simulink model "testboard_UW_GNCDE"  (R2019a)
settings: Solver=FixedStepAuto  StartTime=0.0  StopTime=100  FixedStep=0.05  RelTol=1e-3
values from neighbouring files (symbols this model uses):
  D = zeros(6,3)    [MPCController_test.m]
undefined symbols (not defined in the file or in its folder): Continuous, DiscIntNeverNeededParam, MPCController_test, MPCController_testq, Time
libraries: aerolibutil x23, sharedtransform x5, simulink_extras x4, simulink x4, sharedutil x4, ephemeris x3, sb_quatrans x3, ATV_cowell_plus_tides x2, FO_frame_q x2, FO_ang_vel x2, reference_frame_inv_change x2, sb_qua2con x2
(part 1 of 3)
settings Model: Creator=Jeong miri  LastModifiedBy=Jeong miri
settings SolverCC: AlgebraicLoopSolver=LineSearch
settings DataIOCC: ReturnWorkspaceOutputs=off
settings DebuggingCC: ArithmeticOperatorsInVariantConditions=warning
settings SFSimCC: SimUseLocalCustomCode=off
settings RTWCC: RTWUseLocalCustomCode=off

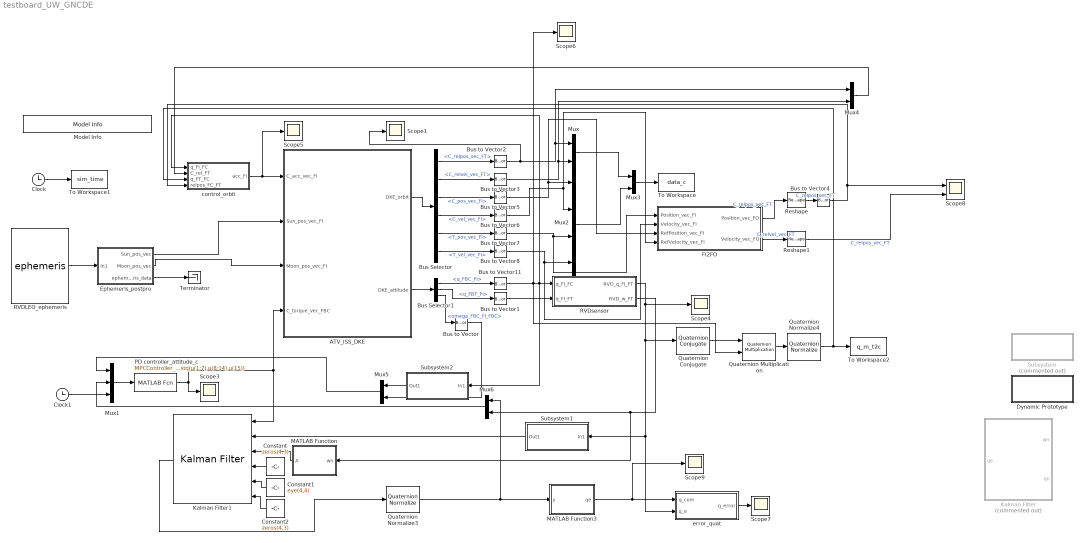
== system testboard_UW_GNCDE ==
  ATV_ISS_DKE : Subsystem
  Bus Selector : BusSelector  OutputSignals=C_relpos_vec_FT,C_relvel_vec_FT,C_pos_vec_FI,C_vel_vec_FI,T_pos_vec_FI,T_vel_vec_FI
  Bus Selector1 : BusSelector  OutputSignals=q_FBC_FI,q_FBT_FI,omega_FBC_FI_FBC
  Bus to Vector{,1..8,11} (10 alike) : BusToVector
  Clock : Clock
  Clock1 : Clock
  Constant : Constant  Value=zeros(4,3)
  Constant1 : Constant  Value=eye(4,4)
  Constant2 : Constant  Value=zeros(4,3)
  Dynamic Prototype : Subsystem
  Ephemeris_postpro : Subsystem
  FI2FO : Subsystem  AncestorBlock=FI_2_FO/FI2FO
  Kalman Filter : Subsystem  Commented=on
  Kalman Filter1 : ctrlSharedLib/Kalman Filter  TimeDomain=Continuous-Time  UseCurrentEstimator=on  ModelSource=Input port  ModelSourceVariable=ss(0.95,1,1,0,1)  A=0.95  B=zeros(3,3)  C=eye(3,3)  D=zeros(3,3)  NumberOfStates=4  NumberOfInputs=3  NumberOfOutputs=4  InitialEstimateSource=Dialog  X0=[0.2685;-0.1449;0.1277;0.9437]  P0=1*eye(4)  UseK=off  UseGH=on  NumberOfProcessNoiseInputs=1  G=eye(4)  TimeInvariantG=on  H=eye(4)  TimeInvariantH=on  Q=(0.25^2)*eye(4)  TimeInvariantQ=on  R=5*eye(4)  TimeInvariantR=on  N=0  TimeInvariantN=on  AddInputPort=on  AddEnablePort=off  OutputEstimatedY=off  OutputP=off  Ts=0.05
      settings: SourceProductBaseCode=CT
  MATLAB Function : MATLAB Function  TreatAsAtomicUnit=on
  MATLAB Function3 : MATLAB Function  TreatAsAtomicUnit=on
  Model Info : simulink/Model-Wide Utilities/Model Info  Frame=on  DisplayStringWithTags=using matlab quaternion formation [1 0 0 0]  HorizontalTextAlignment=Center  LeftAlignmentValue=0.5
  Mux{,3..6} (5 alike) : Mux  Inputs=2
  Mux1 : Mux  Inputs=3
  Mux2 : Mux
  PD controller_attitude_c : MATLABFcn  MATLABFcn=MPCController_testq(u(1:7),u(8:14),u(15))  OutputDimensions=3
  Quaternion Conjugate : aerolibutil/Quaternion Conjugate
      settings: SourceProductName=Aerospace Blockset  SourceProductBaseCode=AE
  Quaternion Multiplication : aerolibutil/Quaternion Multiplication
  Quaternion Normalize3 : sharedutil/Quaternion Normalize  aMode=aMode
      settings: SourceProductName=Aerospace Blockset  SourceProductBaseCode=AE
  Quaternion Normalize4 : sharedutil/Quaternion Normalize  aMode=aMode
      settings: SourceProductName=Aerospace Blockset  SourceProductBaseCode=AE
  RVDLEO_ephemeris : ephemeris/ephemeris  DiagCtrlNo=6  Ini_option=Specify via M-File  InitFileName=D:\GNCDE\working_folder\RVDLEO_ephemeris_init.m  NewFile_Action=Cancel  OldFile_Action=Cancel  InitStatus=on  Ini_Epoch=5479  Enable_Body=[0 0 1 0 0 0 0 0 0 1 1 0 0]  chbycf=struct('EAR',[5474.0194925278993 5479.6117378982699 10 -19525649687.250961 -7242210690.4189663 12591507.829688819 712045.59300004842 -4605.6625453254146 219.47025289226869 7.4245048250737691 -1.279428349516061 0.125436043400523 -0.0071881873469209229 -0.001528338274485566 133532390146.9698 -921020264.59608769 -81156138.833497182 137258.18726933541 1958.221018748188 -226.45025145371531 19.04438678085301 -0.47565199325122492 -0.029635518085251819 0.013715571797866871 -0.0013136744370657459 57865920681.460564 -399022325.11280107 -35186655.777805582 54285.092220920029 985.14747069403722 -69.615781388512403 6.5400659798170437 -0.19345718613262849 -0.0066813954077421999 0.0044218866970717188 -0.00045458987392305651;5479.6117378982699 5485.4983119723438 10 -34254548400.29591 -7477438242.8778076 23337177.440669671 787909.51370320341 -101.42364834386559 199.86116801645741 -13.88804847021297 -0.4553042858772216 0.078328146498667775 0.0059646795681814746 -0.0010337031674248431 130955284596.13721 -1663171194.276058 -87925053.51922065 179251.61568709169 1388.5831853938671 132.30829303924551 9.512894879359461 -1.0347453844758461 -0.041263310503606522 0.0060887801194377117 0.00052000420269988521 56749025379.978554 -720980819.72698534 -38162991.360703968 77270.96408691231 1016.182799768875 49.167254600843748 2.8008634855034802 -0.35644771507836259 -0.011929311143635459 0.0022070878965816838 0.00014552259262877749;5485.4983119723438 5491.3848860464177 10 -48992679504.172363 -7252760915.1633511 32857451.614941169 801439.50634623843 1101.8143140951399 0.083647783492835262 3.9255766985739471 0.82019475446432044 -0.061798440081102357 -0.0061011152711196162 -0.0002389289953963916 126932773131.94701 -2357357426.2140589 -85540006.044280127 225511.99280920179 4182.0883657711947 88.662679826200574 -3.5479097565355282 0.81152795017696377 0.087199738015311973 -0.001151144659435246 -0.00017101715215852651 55004945370.370369 -1022217299.01609 -37102806.967740543 101895.7725987231 1971.0960883287471 28.70521160977616 -1.140951709445895 0.29051978417011931 0.027717464636542951 -0.00048242776422865698 -6.6677991161821385e-05;5491.3848860464177 5497.2714601204916 10 -63204647068.536743 -6951087933.3918591 42601686.903376661 824699.35841737944 1649.568043720418 -113.1790852983782 -41.022970444021972 -4.3406011450349444 0.070110924116653137 0.065367019483753938 0.0058988188212964988 121543214792.2896 -3029554236.4885492 -82357371.525249705 313732.82557588391 7943.5635573665686 408.7545116397921 18.400097415110199 -2.7277057817587891 -0.57221163955953691 -0.023246325824219521 0.0053081507161301267 52667973121.656143 -1313559489.3725569 -35666051.661055617 140488.6937452509 3215.2116641950338 132.83967448087751 5.289527673086579 -0.99991985655036242 -0.18955929431432891 -0.0063908294139869226 0.0019201328415656251;5497.2714601204916 5503.1580341945655 10 -76734737558.20166 -6570839091.8005066 52372771.716799781 772018.39095029037 -9944.6279617588989 -454.3681787485454 83.809068685693589 3.7919618233988972 -1.361770299950025 -0.026622466649221209 0.02451221935319188 114839053481.6221 -3670661103.2674298 -77618855.18230474 479784.41825950157 8682.2149673298591 -705.09161127909567 -38.806502953602752 9.8568103129389719 0.33397462270782607 -0.1701515171819207 -0.001317018702844246 49761592296.068863 -1591106544.9909611 -33607749.850501142 203098.60049911449 3197.4313406917122 -245.8172029376731 -11.19376541302562 3.3690215861258581 0.082996134226937704 -0.057386373093671249 7.2266565342218286e-05;5503.1580341945655 5509.3389369723436 10 -89729309568.452377 -6410491164.686923 67105136.35983476 721521.72513387376 -6928.6403657680194 432.94267085107168 -22.126363115256549 0.072413118060123932 0.30426059359918167 -0.049301053495564191 0.0024480440664662729 106675048463.05949 -4495427655.7620573 -78608325.722655028 606054.10099249275 -537.49477693948893 -26.30040712632232 24.681564052482059 -3.2413175158506959 0.26932602498584729 0.01063421455686926 -0.0051067636571243587 ...(+3004 chars)],'MOO',[5476.6131248693891 5481.114976721241 10 235949301.9451361 -139173673.45685661 -17032226.23224216 1771368.5992196151 71835.615581327787 -7540.910793108279 16.28634176898839 8.9471108610484045 -0.075149790432813265 0.073741168648467623 -0.0079991516308435175 252854781.41849309 127527608.8909824 -17736229.67664988 -1273994.0397991559 120401.39664943211 2097.2510112104869 -328.06212638437131 5.2330344486417859 -0.36780970941805829 0.045648828645552642 0.0054088502705201902 90789604.575848266 39511416.746048398 -6353352.9079350522 -382773.30564623408 41969.292298044027 508.7589280098282 -108.8642852811857 1.9853812338043171 -0.12726475804964901 0.017146034811725702 0.0016172965508710921;5481.114976721241 5486.0260878323525 10 -119281955.3483213 -194445073.75190681 8804733.5933451802 2314797.0242647119 -80112.933901338925 -5728.0071634057631 421.759363826666 -0.91181921354713247 -1.9488246940505889 -0.0084783699209460186 0.011503361945009101 333270850.53264862 -53856696.543870591 -24894022.82772788 876282.02549440751 131553.5833390374 -5694.0238152214242 -120.8246642842264 26.977974360037859 -0.069136334149162204 -0.1355218644754167 -0.00041516536287204377 109482735.19933949 -22556141.111693509 -8127972.0992596922 347532.41299178731 41893.033387395917 -2039.8857338279649 -29.532861950791968 8.9895693748721577 -0.069175183404102503 -0.0454504927427863 0.00013279297195722601;5486.0260878323525 5491.1418285730924 10 -368209659.5822103 -37272448.254160039 28966093.382118989 575792.99784778652 -147195.65970897651 -1320.7880421427931 -160.4890923653515 -24.126983670689832 1.796771915897017 0.1446034638555122 0.0033626189383728958 71454414.966571927 -191741260.26137051 -5312399.1746770367 2402447.2617379432 37282.834321171671 -3936.0102596018878 106.2381311707356 -27.158974243902669 -2.3056748101124969 0.036254948464378732 0.0017252666010675959 16003973.15075887 -65111328.583141513 -1125438.4316383279 814225.58604786242 8984.5804238699893 -1322.8460257668189 32.849456061550768 -9.6427815500062568 -0.72953118229025593 0.01518347286777523 0.00062416681064214065;5491.1418285730924 5495.8483100545745 10 -236519463.35481861 158989676.51849779 17929698.965212502 -1637619.3726077219 -148555.9306766433 -1013.984913001647 511.68040453812893 71.721969906101265 2.6806624200266191 -0.32312680059878268 -0.051766975946830517 -254997418.9626143 -114164435.1907489 19450237.914976511 1721414.0568385541 -68076.258331813486 -9423.4410594721303 -559.55193870543053 6.4195501401895942 5.5801097229978307 0.44785715250136943 -0.00073204452341000007 -90573889.219337761 -34836986.375739031 6887264.9110708293 538411.5582076998 -25810.146240520378 -3153.833007474484 -176.40199327653519 3.6184785576243348 1.918418425226208 0.14277676416418511 -0.001316420239122922;5495.8483100545745 5499.9409026471667 10 116401656.6447359 171813227.58897761 -7970534.7329276307 -1980863.751555094 25524.273659049239 11206.54795115962 167.1969016831396 -69.268389378915458 -3.278822889780431 0.47172691310630382 0.041157636499332413 -303323196.63847512 65757614.980408177 20611242.479798179 -543872.05192871974 -143426.6800424523 -92.085434493212006 813.24375163807758 25.531789254040699 -5.4093457119175339 -0.35587524108731272 0.036090681683312989 -99338439.864302963 25569036.202503979 6717133.6882401844 -223199.74185484409 -47253.39209144537 203.64275772509021 274.67240678849907 7.0777808184736957 -1.873842176894027 -0.1089760039254066 0.012906262764400741;5499.9409026471667 5504.2381248693891 10 335274982.68933171 31989042.783745591 -25328830.028744549 -162112.32263660929 178384.79872649111 -3587.6855037252139 -820.42089911496646 65.820233209958843 2.5672242334859812 -0.70311518487965996 0.016015888366578648 -42449594.014380872 180569964.27288741 3160527.406108255 -2220172.1798197869 10148.981021424101 11731.155453871979 -511.53838286409859 -48.826068979201182 6.727900076266061 0.040477776788079907 -0.062120147956740618 -7587826.408630427 61015956.372747831 534922.55756132503 ...(+4277 chars)],'SUN',[5478.8683078666654 5482.1318495333317 10 425902245.7615025 967998.27965419751 -617.75881662588279 0.45980846342291071 -0.0043364422167170577 -0.00020171772762461309 -1.225011122694448e-05 2.3865395757416262e-05 -2.9291117847822658e-07 -1.4546880485764169e-05 1.7380347169454301e-06 -108117502.82189821 1184470.971916039 573.98858879357738 0.81449435548467708 0.0123702264478636 0.00013669158135858479 3.0125458983458141e-06 2.1288618992704241e-05 -6.7756159307572082e-07 -1.403173841314433e-05 -1.857921382276252e-07 -69272546.646467105 487629.54570443952 253.7339345238355 0.32242200756521211 0.0068109215496674307 9.5519179459789061e-05 2.1833006097486991e-06 8.3557192063880096e-06 -2.1110260248094199e-07 -5.6051094059912039e-06 -2.0946789385142999e-07;5482.1318495333317 5485.3953911999988 10 427833316.66130322 963076.75062086084 -612.81277980640903 0.35080907664054523 -0.0098922992050331573 -0.00036380103125100522 3.4787407022091389e-05 -2.2510980377448619e-05 1.3232521644046419e-05 7.1238643550083942e-06 -2.365423327018569e-05 -105743935.5028107 1189105.5542703699 585.04217680491035 1.034374393213618 0.01494844902950113 0.0001128347597781029 4.9527524415888863e-05 -2.7796809432373019e-05 1.630835977050129e-05 8.7087311958026212e-06 -2.9201894700000078e-05 -68295244.023768201 489676.8979657052 258.32295275562421 0.4474318438385767 0.0087913834942875291 9.881859481749497e-05 2.0776569270259942e-05 -1.145538201128545e-05 6.7149878235458709e-06 3.5807508913316201e-06 -1.202574834275584e-05;5485.3953911999988 5488.6589328666651 10 429754578.667633 958187.74978908116 -609.83857615235684 0.1205345604510957 -0.01960343183724023 -0.0006127452198189477 -7.9062290558582653e-06 2.74258294033769e-05 1.048152071636293e-08 -3.1105645691112532e-06 -2.4413683898238059e-08 -103361001.81192879 1193839.709181759 598.92989905955869 1.281004497556963 0.015222974588530161 -0.00013087953892676479 -1.332699415056042e-05 3.3566256858805422e-05 2.6492958013671179e-08 -3.8929222441107083e-06 7.5831507774073641e-09 -67313804.871897265 491767.47291078261 264.58809424093681 0.5997629617568967 0.0099732697458197843 -3.9234019734949669e-06 -6.2909046714770183e-06 1.375544700613195e-05 9.0153124803999111e-09 -1.602243585618814e-06 3.9688172474391426e-09;5488.6589328666651 5491.9224745333322 10 431666075.64912122 953308.54272034869 -610.69050058190032 -0.29522001779436791 -0.032560179185275713 -0.00063769216996900548 -3.7568219444939769e-05 -2.1232867197447911e-05 -1.31233059770635e-05 6.9470684537333863e-06 2.3502008073023108e-05 -100968479.5393621 1198696.487966035 615.62772922950217 1.486703382835258 0.0090890481669985458 -0.00052773820111920303 -7.6513213257555648e-05 -2.7940788477935931e-05 -1.6522110177634789e-05 8.7957053984471832e-06 2.9504452827943529e-05 -66328128.548470423 493915.62540751451 272.71440034669598 0.74993844429844181 0.0080708103200663774 -0.00021479404065349211 -3.4810126893800589e-05 -1.16192723079181e-05 -6.8050026633825354e-06 3.6294036247714051e-06 1.2152612474318969e-05;5491.9224745333322 5495.1860161999984 10 433567789.14228028 948399.08975899057 -617.74216249937842 -0.90443727124774398 -0.042150143336950122 -0.00020611852235782809 3.3006234403551652e-05 1.889243790533144e-05 1.7957531259145181e-08 -1.170322464091036e-05 -9.584396314881587e-09 -98566103.968162954 1203694.325045964 633.88697057074683 1.5162833821050461 -0.006986482396130706 -0.001041627972896495 -1.454473517768674e-05 2.3530468906999719e-05 4.2635722420597832e-08 -1.489176693246279e-05 -1.008424931208629e-08 -65338085.827350713 496135.08493469068 282.28695978902317 0.8266120414065431 0.00051181247966610105 -0.00053298136502892286 -1.11527811599427e-05 9.6900546132360124e-06 2.5843636673005951e-08 -6.1363848759836404e-06 -8.9783050194230303e-09;5495.1860161999984 5498.4495578666656 10 435459602.91844511 943402.28254764038 -632.61679142927665 -1.5615545107120801 -0.036837430038632289 0.00078284486666512529 7.6408705632018858e-05 -1.2745567518235389e-05 ...(+8142 chars)],'MER',[0 0 0 0 0 0 0 0 0 0 0 0 0 0 0 0 0 0 0 0 0 0 0 0 0 0 0 0 0 0 0 0 0 0 0 0;0 0 0 0 0 0 0 0 0 0 0 0 0 0 0 0 0 0 0 0 0 0 0 0 0 0 0 0 0 0 0 0 0 0 0 0;0 0 0 0 0 0 0 0 0 0 0 0 0 0 0 0 0 0 0 0 0 0 0 0 0 0 0 0 0 0 0 0 0 0 0 0;0 0 0 0 0 0 0 0 0 0 0 0 0 0 0 0 0 0 0 0 0 0 0 0 0 0 0 0 0 0 0 0 0 0 0 0;0 0 0 0 0 0 0 0 0 0 0 0 0 0 0 0 0 0 0 0 0 0 0 0 0 0 0 0 0 0 0 0 0 0 0 0;0 0 0 0 0 0 0 0 0 0 0 0 0 0 0 0 0 0 0 0 0 0 0 0 0 0 0 0 0 0 0 0 0 0 0 0;0 0 0 0 0 0 0 0 0 0 0 0 0 0 0 0 0 0 0 0 0 0 0 0 0 0 0 0 0 0 0 0 0 0 0 0;0 0 0 0 0 0 0 0 0 0 0 0 0 0 0 0 0 0 0 0 0 0 0 0 0 0 0 0 0 0 0 0 0 0 0 0;0 0 0 0 0 0 0 0 0 0 0 0 0 0 0 0 0 0 0 0 0 0 0 0 0 0 0 0 0 0 0 0 0 0 0 0;0 0 0 0 0 0 0 0 0 0 0 0 0 0 0 0 0 0 0 0 0 0 0 0 0 0 0 0 0 0 0 0 0 0 0 0],'VEN',[0 0 0 0 0 0 0 0 0 0 0 0 0 0 0 0 0 0 0 0 0 0 0 0 0 0 0 0 0 0 0 0 0 0 0 0;0 0 0 0 0 0 0 0 0 0 0 0 0 0 0 0 0 0 0 0 0 0 0 0 0 0 0 0 0 0 0 0 0 0 0 0;0 0 0 0 0 0 0 0 0 0 0 0 0 0 0 0 0 0 0 0 0 0 0 0 0 0 0 0 0 0 0 0 0 0 0 0;0 0 0 0 0 0 0 0 0 0 0 0 0 0 0 0 0 0 0 0 0 0 0 0 0 0 0 0 0 0 0 0 0 0 0 0;0 0 0 0 0 0 0 0 0 0 0 0 0 0 0 0 0 0 0 0 0 0 0 0 0 0 0 0 0 0 0 0 0 0 0 0;0 0 0 0 0 0 0 0 0 0 0 0 0 0 0 0 0 0 0 0 0 0 0 0 0 0 0 0 0 0 0 0 0 0 0 0;0 0 0 0 0 0 0 0 0 0 0 0 0 0 0 0 0 0 0 0 0 0 0 0 0 0 0 0 0 0 0 0 0 0 0 0;0 0 0 0 0 0 0 0 0 0 0 0 0 0 0 0 0 0 0 0 0 0 0 0 0 0 0 0 0 0 0 0 0 0 0 0;0 0 0 0 0 0 0 0 0 0 0 0 0 0 0 0 0 0 0 0 0 0 0 0 0 0 0 0 0 0 0 0 0 0 0 0;0 0 0 0 0 0 0 0 0 0 0 0 0 0 0 0 0 0 0 0 0 0 0 0 0 0 0 0 0 0 0 0 0 0 0 0],'MAR',[0 0 0 0 0 0 0 0 0 0 0 0 0 0 0 0 0 0 0 0 0 0 0 0 0 0 0 0 0 0 0 0 0 0 0 0;0 0 0 0 0 0 0 0 0 0 0 0 0 0 0 0 0 0 0 0 0 0 0 0 0 0 0 0 0 0 0 0 0 0 0 0;0 0 0 0 0 0 0 0 0 0 0 0 0 0 0 0 0 0 0 0 0 0 0 0 0 0 0 0 0 0 0 0 0 0 0 0;0 0 0 0 0 0 0 0 0 0 0 0 0 0 0 0 0 0 0 0 0 0 0 0 0 0 0 0 0 0 0 0 0 0 0 0;0 0 0 0 0 0 0 0 0 0 0 0 0 0 0 0 0 0 0 0 0 0 0 0 0 0 0 0 0 0 0 0 0 0 0 0;0 0 0 0 0 0 0 0 0 0 0 0 0 0 0 0 0 0 0 0 0 0 0 0 0 0 0 0 0 0 0 0 0 0 0 0;0 0 0 0 0 0 0 0 0 0 0 0 0 0 0 0 0 0 0 0 0 0 0 0 0 0 0 0 0 0 0 0 0 0 0 0;0 0 0 0 0 0 0 0 0 0 0 0 0 0 0 0 0 0 0 0 0 0 0 0 0 0 0 0 0 0 0 0 0 0 0 0;0 0 0 0 0 0 0 0 0 0 0 0 0 0 0 0 0 0 0 0 0 0 0 0 0 0 0 0 0 0 0 0 0 0 0 0;0 0 0 0 0 0 0 0 0 0 0 0 0 0 0 0 0 0 0 0 0 0 0 0 0 0 0 0 0 0 0 0 0 0 0 0],'JUP',[0 0 0 0 0 0 0 0 0 0 0 0 0 0 0 0 0 0 0 0 0 0 0 0 0 0 0 0 0 0 0 0 0 0 0 0;0 0 0 0 0 0 0 0 0 0 0 0 0 0 0 0 0 0 0 0 0 0 0 0 0 0 0 0 0 0 0 0 0 0 0 0;0 0 0 0 0 0 0 0 0 0 0 0 0 0 0 0 0 0 0 0 0 0 0 0 0 0 0 0 0 0 0 0 0 0 0 0;0 0 0 0 0 0 0 0 0 0 0 0 0 0 0 0 0 0 0 0 0 0 0 0 0 0 0 0 0 0 0 0 0 0 0 0;0 0 0 0 0 0 0 0 0 0 0 0 0 0 0 0 0 0 0 0 0 0 0 0 0 0 0 0 0 0 0 0 0 0 0 0;0 0 0 0 0 0 0 0 0 0 0 0 0 0 0 0 0 0 0 0 0 0 0 0 0 0 0 0 0 0 0 0 0 0 0 0;0 0 0 0 0 0 0 0 0 0 0 0 0 0 0 0 0 0 0 0 0 0 0 0 0 0 0 0 0 0 0 0 0 0 0 0;0 0 0 0 0 0 0 0 0 0 0 0 0 0 0 0 0 0 0 0 0 0 0 0 0 0 0 0 0 0 0 0 0 0 0 0;0 0 0 0 0 0 0 0 0 0 0 0 0 0 0 0 0 0 0 0 0 0 0 0 0 0 0 0 0 0 0 0 0 0 0 0;0 0 0 0 0 0 0 0 0 0 0 0 0 0 0 0 0 0 0 0 0 0 0 0 0 0 0 0 0 0 0 0 0 0 0 0],'SAT',[0 0 0 0 0 0 0 0 0 0 0 0 0 0 0 0 0 0 0 0 0 0 0 0 0 0 0 0 0 0 0 0 0 0 0 0;0 0 0 0 0 0 0 0 0 0 0 0 0 0 0 0 0 0 0 0 0 0 0 0 0 0 0 0 0 0 0 0 0 0 0 0;0 0 0 0 0 0 0 0 0 0 0 0 0 0 0 0 0 0 0 0 0 0 0 0 0 0 0 0 0 0 0 0 0 0 0 0;0 0 0 0 0 0 0 0 0 0 0 0 0 0 0 0 0 0 0 0 0 0 0 0 0 0 0 0 0 0 0 0 0 0 0 0;0 0 0 0 0 0 0 0 0 0 0 0 0 0 0 0 0 0 0 0 0 0 0 0 0 0 0 0 0 0 0 0 0 0 0 0;0 0 0 0 0 0 0 0 0 0 0 0 0 0 0 0 0 0 0 0 0 0 0 0 0 0 0 0 0 0 0 0 0 0 0 0;0 0 0 0 0 0 0 0 0 0 0 0 0 0 0 0 0 0 0 0 0 0 0 0 0 0 0 0 0 0 0 0 0 0 0 0;0 0 0 0 0 0 0 0 0 0 0 0 0 0 0 0 0 0 0 0 0 0 0 0 0 0 0 0 0 0 0 0 0 0 0 0;0 0 0 0 0 0 0 0 0 0 0 0 0 0 0 0 0 0 0 0 0 0 0 0 0 0 0 0 0 0 0 0 0 0 0 0;0 0 0 0 0 0 0 0 0 0 0 0 0 0 0 0 0 0 0 0 0 0 0 0 0 0 0 0 0 0 0 0 0 0 0 0],'URA',[0 0 0 0 0 0 0 0 0 0 0 0 0 0 0 0 0 0 0 0 0 0 0 0 0 0 0 0 0 0 0 0 0 0 0 0;0 0 0 0 0 0 0 0 0 0 0 0 0 0 0 0 0 0 0 0 0 0 0 0 0 0 0 0 0 0 0 0 0 0 0 0;0 0 0 0 0 0 0 0 0 0 0 0 0 0 0 0 0 0 0 0 0 0 0 0 0 0 0 0 0 0 0 0 0 0 0 0;0 0 0 0 0 0 0 0 0 0 0 0 0 0 0 0 0 0 0 0 0 0 0 0 0 0 0 0 0 0 0 0 0 0 0 0;0 0 0 0 0 0 0 0 0 0 0 0 0 0 0 0 0 0 0 0 0 0 0 0 0 0 0 0 0 0 0 0 0 0 0 0;0 0 0 0 0 0 0 0 0 0 0 0 0 0 0 0 0 0 0 0 0 0 0 0 0 0 0 0 0 0 0 0 0 0 0 0;0 0 0 0 0 0 0 0 0 0 0 0 0 0 0 0 0 0 0 0 0 0 0 0 0 0 0 0 0 0 0 0 0 0 0 0;0 0 0 0 0 0 0 0 0 0 0 0 0 0 0 0 0 0 0 0 0 0 0 0 0 0 0 0 0 0 0 0 0 0 0 0;0 0 0 0 0 0 0 0 0 0 0 0 0 0 0 0 0 0 0 0 0 0 0 0 0 0 0 0 0 0 0 0 0 0 0 0;0 0 0 0 0 0 0 0 0 0 0 0 0 0 0 0 0 0 0 0 0 0 0 0 0 0 0 0 0 0 0 0 0 0 0 0],'NEP',[0 0 0 0 0 0 0 0 0 0 0 0 0 0 0 0 0 0 0 0 0 0 0 0 0 0 0 0 0 0 0 0 0 0 0 0;0 0 0 0 0 0 0 0 0 0 0 0 0 0 0 0 0 0 0 0 0 0 0 0 0 0 0 0 0 0 0 0 0 0 0 0;0 0 0 0 0 0 0 0 0 0 0 0 0 0 0 0 0 0 0 0 0 0 0 0 0 0 0 0 0 0 0 0 0 0 0 0;0 0 0 0 0 0 0 0 0 0 0 0 0 0 0 0 0 0 0 0 0 0 0 0 0 0 0 0 0 0 0 0 0 0 0 0;0 0 0 0 0 0 0 0 0 0 0 0 0 0 0 0 0 0 0 0 0 0 0 0 0 0 0 0 0 0 0 0 0 0 0 0;0 0 0 0 0 0 0 0 0 0 0 0 0 0 0 0 0 0 0 0 0 0 0 0 0 0 0 0 0 0 0 0 0 0 0 0;0 0 0 0 0 0 0 0 0 0 0 0 0 0 0 0 0 0 0 0 0 0 0 0 0 0 0 0 0 0 0 0 0 0 0 0;0 0 0 0 0 0 0 0 0 0 0 0 0 0 0 0 0 0 0 0 0 0 0 0 0 0 0 0 0 0 0 0 0 0 0 0;0 0 0 0 0 0 0 0 0 0 0 0 0 0 0 0 0 0 0 0 0 0 0 0 0 0 0 0 0 0 0 0 0 0 0 0;0 0 0 0 0 0 0 0 0 0 0 0 0 0 0 0 0 0 0 0 0 0 0 0 0 0 0 0 0 0 0 0 0 0 0 0],'PLU',[0 0 0 0 0 0 0 0 0 0 0 0 0 0 0 0 0 0 0 0 0 0 0 0 0 0 0 0 0 0 0 0 0 0 0 0;0 0 0 0 0 0 0 0 0 0 0 0 0 0 0 0 0 0 0 0 0 0 0 0 0 0 0 0 0 0 0 0 0 0 0 0;0 0 0 0 0 0 0 0 0 0 0 0 0 0 0 0 0 0 0 0 0 0 0 0 0 0 0 0 0 0 0 0 0 0 0 0;0 0 0 0 0 0 0 0 0 0 0 0 0 0 0 0 0 0 0 0 0 0 0 0 0 0 0 0 0 0 0 0 0 0 0 0;0 0 0 0 0 0 0 0 0 0 0 0 0 0 0 0 0 0 0 0 0 0 0 0 0 0 0 0 0 0 0 0 0 0 0 0;0 0 0 0 0 0 0 0 0 0 0 0 0 0 0 0 0 0 0 0 0 0 0 0 0 0 0 0 0 0 0 0 0 0 0 0;0 0 0 0 0 0 0 0 0 0 0 0 0 0 0 0 0 0 0 0 0 0 0 0 0 0 0 0 0 0 0 0 0 0 0 0;0 0 0 0 0 0 0 0 0 0 0 0 0 0 0 0 0 0 0 0 0 0 0 0 0 0 0 0 0 0 0 0 0 0 0 0;0 0 0 0 0 0 0 0 0 0 0 0 0 0 0 0 0 0 0 0 0 0 0 0 0 0 0 0 0 0 0 0 0 0 0 0;0 0 0 0 0 0 0 0 0 0 0 0 0 0 0 0 0 0 0 0 0 0 0 0 0 0 0 0 0 0 0 0 0 0 0 0],'PHO',[0 0 0 0 0 0 0 0 0 0 0 0 0 0 0 0 0 0 0 0 0 0 0 0 0 0 0 0 0 0 0 0 0 0 0 0;0 0 0 0 0 0 0 0 0 0 0 0 0 0 0 0 0 0 0 0 0 0 0 0 0 0 0 0 0 0 0 0 0 0 0 0;0 0 0 0 0 0 0 0 0 0 0 0 0 0 0 0 0 0 0 0 0 0 0 0 0 0 0 0 0 0 0 0 0 0 0 0;0 0 0 0 0 0 0 0 0 0 0 0 0 0 0 0 0 0 0 0 0 0 0 0 0 0 0 0 0 0 0 0 0 0 0 0;0 0 0 0 0 0 0 0 0 0 0 0 0 0 0 0 0 0 0 0 0 0 0 0 0 0 0 0 0 0 0 0 0 0 0 0;0 0 0 0 0 0 0 0 0 0 0 0 0 0 0 0 0 0 0 0 0 0 0 0 0 0 0 0 0 0 0 0 0 0 0 0;0 0 0 0 0 0 0 0 0 0 0 0 0 0 0 0 0 0 0 0 0 0 0 0 0 0 0 0 0 0 0 0 0 0 0 0;0 0 0 0 0 0 0 0 0 0 0 0 0 0 0 0 0 0 0 0 0 0 0 0 0 0 0 0 0 0 0 0 0 0 0 0;0 0 0 0 0 0 0 0 0 0 0 0 0 0 0 0 0 0 0 0 0 0 0 0 0 0 0 0 0 0 0 0 0 0 0 0;0 0 0 0 0 0 0 0 0 0 0 0 0 0 0 0 0 0 0 0 0 0 0 0 0 0 0 0 0 0 0 0 0 0 0 0],'DEI',[0 0 0 0 0 0 0 0 0 0 0 0 0 0 0 0 0 0 0 0 0 0 0 0 0 0 0 0 0 0 0 0 0 0 0 0;0 0 0 0 0 0 0 0 0 0 0 0 0 0 0 0 0 0 0 0 0 0 0 0 0 0 0 0 0 0 0 0 0 0 0 0;0 0 0 0 0 0 0 0 0 0 0 0 0 0 0 0 0 0 0 0 0 0 0 0 0 0 0 0 0 0 0 0 0 0 0 0;0 0 0 0 0 0 0 0 0 0 0 0 0 0 0 0 0 0 0 0 0 0 0 0 0 0 0 0 0 0 0 0 0 0 0 0;0 0 0 0 0 0 0 0 0 0 0 0 0 0 0 0 0 0 0 0 0 0 0 0 0 0 0 0 0 0 0 0 0 0 0 0;0 0 0 0 0 0 0 0 0 0 0 0 0 0 0 0 0 0 0 0 0 0 0 0 0 0 0 0 0 0 0 0 0 0 0 0;0 0 0 0 0 0 0 0 0 0 0 0 0 0 0 0 0 0 0 0 0 0 0 0 0 0 0 0 0 0 0 0 0 0 0 0;0 0 0 0 0 0 0 0 0 0 0 0 0 0 0 0 0 0 0 0 0 0 0 0 0 0 0 0 0 0 0 0 0 0 0 0;0 0 0 0 0 0 0 0 0 0 0 0 0 0 0 0 0 0 0 0 0 0 0 0 0 0 0 0 0 0 0 0 0 0 0 0;0 0 0 0 0 0 0 0 0 0 0 0 0 0 0 0 0 0 0 0 0 0 0 0 0 0 0 0 0 0 0 0 0 0 0 0])
  RVDsensor : Subsystem
  Reshape : Reshape
  Reshape1 : Reshape
  Scope{1,3..7,9} (7 alike) : Scope
  Scope8 : Scope  NumInputPorts=2
  Subsystem : Subsystem  Commented=on
  Subsystem1 : Subsystem
  Subsystem2 : Subsystem
  Terminator : Terminator
  To Workspace : ToWorkspace  VariableName=data_c  SampleTime=-1
  To Workspace1 : ToWorkspace  VariableName=sim_time  SampleTime=-1
  To Workspace2 : ToWorkspace  VariableName=q_m_t2c  SaveFormat=Timeseries  SampleTime=-1
  control_orbit : Subsystem
  error_quat : Subsystem
  wires:
  Ephemeris_postpro/3(ephemeris_data) -> Terminator/1
  Ephemeris_postpro/2(Moon_pos_vec) -> ATV_ISS_DKE/3(Moon_pos_vec_FI)
  Ephemeris_postpro/1(Sun_pos_vec) -> ATV_ISS_DKE/2(Sun_pos_vec_FI)
  RVDLEO_ephemeris/1 -> Ephemeris_postpro/1(In1)
  ATV_ISS_DKE/1(DKE_orbit) -> Bus Selector/1
  Bus Selector/1 -> Bus to Vector2/1  "<C_relpos_vec_FT>"
  Bus Selector/2 -> Bus to Vector3/1  "<C_relvel_vec_FT>"
  ATV_ISS_DKE/2(DKE_attitude) -> Bus Selector1/1
  Bus Selector1/1 -> Bus to Vector11/1  "<q_FBC_FI>"
  Bus Selector1/2 -> Bus to Vector1/1  "<q_FBT_FI>"
  Bus to Vector1/1 -> RVDsensor/2(q_FI_FT)
  Bus to Vector2/1 -> Scope1/1, Mux4/1, Mux/1
  Bus to Vector3/1 -> Mux4/2, Mux/2
  Mux1/1 -> PD controller_attitude_c/1
  Mux/1 -> Mux3/1
  Bus Selector/3 -> Bus to Vector5/1  "<C_pos_vec_FI>"
  Bus Selector/4 -> Bus to Vector6/1  "<C_vel_vec_FI>"
  Bus Selector/5 -> Bus to Vector7/1  "<T_pos_vec_FI>"
  Bus Selector/6 -> Bus to Vector8/1  "<T_vel_vec_FI>"
  Bus to Vector5/1 -> FI2FO/3(RefPosition_vec_FI), Mux2/1
  Bus to Vector6/1 -> FI2FO/4(RefVelocity_vec_FI), Mux2/2
  Bus to Vector7/1 -> FI2FO/1(Position_vec_FI), Mux2/3
  Bus to Vector8/1 -> Mux2/4, FI2FO/2(Velocity_vec_FI)
  Mux2/1 -> Mux3/2
  Mux3/1 -> To Workspace/1
  Clock/1 -> To Workspace1/1
  Mux4/1 -> control_orbit/2(C_rel_FT)
  Bus Selector1/3 -> Bus to Vector/1  "<omega_FBC_FI_FBC>"
  Bus to Vector/1 -> Mux5/2
  Bus to Vector11/1 -> Subsystem2/1(In1), RVDsensor/1(q_FI_FC), control_orbit/1(q_FI_FC), Scope6/1, Quaternion Multiplication/2
  RVDsensor/1(RVD_q_FI_FT) -> Subsystem1/1(In1), error_quat/2(q_e), Quaternion Conjugate/1, Scope4/1
  RVDsensor/2(RVD_w_FT) -> MATLAB Function/1(wn), Mux6/2
  Constant/1 -> Kalman Filter1/4
  MATLAB Function/1(A) -> Kalman Filter1/3
  Constant1/1 -> Kalman Filter1/5
  Subsystem1/1(Out1) -> Kalman Filter1/2
  Constant2/1 -> Kalman Filter1/6
  PD controller_attitude_c/1 -> Kalman Filter1/1, ATV_ISS_DKE/4(C_torque_vec_FBC), Scope3/1
  control_orbit/1(acc_FI) -> Scope5/1, ATV_ISS_DKE/1(C_acc_vec_FI)
  Clock1/1 -> Mux1/3
  Mux5/1 -> Mux1/1
  Mux6/1 -> Mux1/2
  Subsystem2/1(Out1) -> Mux5/1
  error_quat/1(q_error) -> Scope7/1
  Kalman Filter1/1 -> Quaternion Normalize3/1
  Quaternion Normalize3/1 -> Mux6/1, MATLAB Function3/1(y)
  MATLAB Function3/1(qe) -> Scope9/1, error_quat/1(q_com)
  FI2FO/1(Position_vec_FO) -> Reshape/1  "C_relpos_vec_FT"
  FI2FO/2(Velocity_vec_FO) -> Reshape1/1  "C_relvel_vec_FT"
  Reshape/1 -> Bus to Vector4/1  "C_relpos_vec_FT"
  Reshape1/1 -> Scope8/2  "C_relpos_vec_FT"
  Quaternion Conjugate/1 -> Quaternion Multiplication/1
  Quaternion Multiplication/1 -> Quaternion Normalize4/1
  Quaternion Normalize4/1 -> control_orbit/3(q_FT_FC), To Workspace2/1
  Bus to Vector4/1 -> control_orbit/4(relpos_FC_FT), Scope8/1

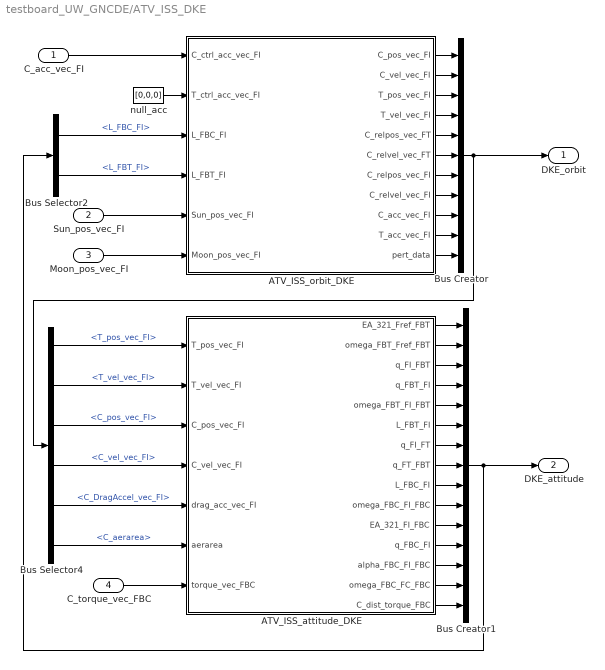
== system testboard_UW_GNCDE/ATV_ISS_DKE ==
  C_acc_vec_FI : Inport
  Sun_pos_vec_FI : Inport  Port=2
  Moon_pos_vec_FI : Inport  Port=3
  C_torque_vec_FBC : Inport  Port=4
  ATV_ISS_attitude_DKE : Subsystem
  ATV_ISS_orbit_DKE : Subsystem
  Bus Creator : BusCreator  Inputs=11
  Bus Creator1 : BusCreator  Inputs=15
  Bus Selector2 : BusSelector  OutputSignals=L_FBC_FI,L_FBT_FI
  Bus Selector4 : BusSelector  OutputSignals=T_pos_vec_FI,T_vel_vec_FI,C_pos_vec_FI,C_vel_vec_FI,pert_data.signal1.C_DragAccel_vec_FI,pert_data.signal1.C_aerarea
  null_acc : Constant  Value=[0,0,0]
  DKE_orbit : Outport
  DKE_attitude : Outport  Port=2
  wires:
  ATV_ISS_orbit_DKE/1(C_pos_vec_FI) -> Bus Creator/1
  ATV_ISS_orbit_DKE/2(C_vel_vec_FI) -> Bus Creator/2
  ATV_ISS_orbit_DKE/3(T_pos_vec_FI) -> Bus Creator/3
  ATV_ISS_orbit_DKE/4(T_vel_vec_FI) -> Bus Creator/4
  ATV_ISS_orbit_DKE/5(C_relpos_vec_FT) -> Bus Creator/5
  ATV_ISS_orbit_DKE/6(C_relvel_vec_FT) -> Bus Creator/6
  ATV_ISS_orbit_DKE/7(C_relpos_vec_FI) -> Bus Creator/7
  ATV_ISS_orbit_DKE/8(C_relvel_vec_FI) -> Bus Creator/8
  ATV_ISS_orbit_DKE/9(C_acc_vec_FI) -> Bus Creator/9
  ATV_ISS_orbit_DKE/10(T_acc_vec_FI) -> Bus Creator/10
  ATV_ISS_orbit_DKE/11(pert_data) -> Bus Creator/11
  ATV_ISS_attitude_DKE/1(EA_321_Fref_FBT) -> Bus Creator1/1
  ATV_ISS_attitude_DKE/2(omega_FBT_Fref_FBT) -> Bus Creator1/2
  ATV_ISS_attitude_DKE/3(q_FI_FBT) -> Bus Creator1/3
  ATV_ISS_attitude_DKE/4(q_FBT_FI) -> Bus Creator1/4
  ATV_ISS_attitude_DKE/5(omega_FBT_FI_FBT) -> Bus Creator1/5
  ATV_ISS_attitude_DKE/6(L_FBT_FI) -> Bus Creator1/6
  ATV_ISS_attitude_DKE/7(q_FI_FT) -> Bus Creator1/7
  ATV_ISS_attitude_DKE/8(q_FT_FBT) -> Bus Creator1/8
  ATV_ISS_attitude_DKE/9(L_FBC_FI) -> Bus Creator1/9
  ATV_ISS_attitude_DKE/10(omega_FBC_FI_FBC) -> Bus Creator1/10
  ATV_ISS_attitude_DKE/11(EA_321_FI_FBC) -> Bus Creator1/11
  ATV_ISS_attitude_DKE/12(q_FBC_FI) -> Bus Creator1/12
  ATV_ISS_attitude_DKE/13(alpha_FBC_FI_FBC) -> Bus Creator1/13
  ATV_ISS_attitude_DKE/14(omega_FBC_FC_FBC) -> Bus Creator1/14
  Bus Creator/1 -> Bus Selector4/1, DKE_orbit/1
  Bus Selector4/1 -> ATV_ISS_attitude_DKE/1(T_pos_vec_FI)  "<T_pos_vec_FI>"
  Bus Selector4/2 -> ATV_ISS_attitude_DKE/2(T_vel_vec_FI)  "<T_vel_vec_FI>"
  Bus Selector4/3 -> ATV_ISS_attitude_DKE/3(C_pos_vec_FI)  "<C_pos_vec_FI>"
  Bus Selector4/4 -> ATV_ISS_attitude_DKE/4(C_vel_vec_FI)  "<C_vel_vec_FI>"
  Bus Selector2/1 -> ATV_ISS_orbit_DKE/3(L_FBC_FI)  "<L_FBC_FI>"
  Bus Selector2/2 -> ATV_ISS_orbit_DKE/4(L_FBT_FI)  "<L_FBT_FI>"
  null_acc/1 -> ATV_ISS_orbit_DKE/2(T_ctrl_acc_vec_FI)
  Sun_pos_vec_FI/1 -> ATV_ISS_orbit_DKE/5(Sun_pos_vec_FI)
  Moon_pos_vec_FI/1 -> ATV_ISS_orbit_DKE/6(Moon_pos_vec_FI)
  Bus Creator1/1 -> Bus Selector2/1, DKE_attitude/1
  C_acc_vec_FI/1 -> ATV_ISS_orbit_DKE/1(C_ctrl_acc_vec_FI)
  C_torque_vec_FBC/1 -> ATV_ISS_attitude_DKE/7(torque_vec_FBC)
  Bus Selector4/5 -> ATV_ISS_attitude_DKE/5(drag_acc_vec_FI)  "<C_DragAccel_vec_FI>"
  Bus Selector4/6 -> ATV_ISS_attitude_DKE/6(aerarea)  "<C_aerarea>"
  ATV_ISS_attitude_DKE/15(C_dist_torque_FBC) -> Bus Creator1/15

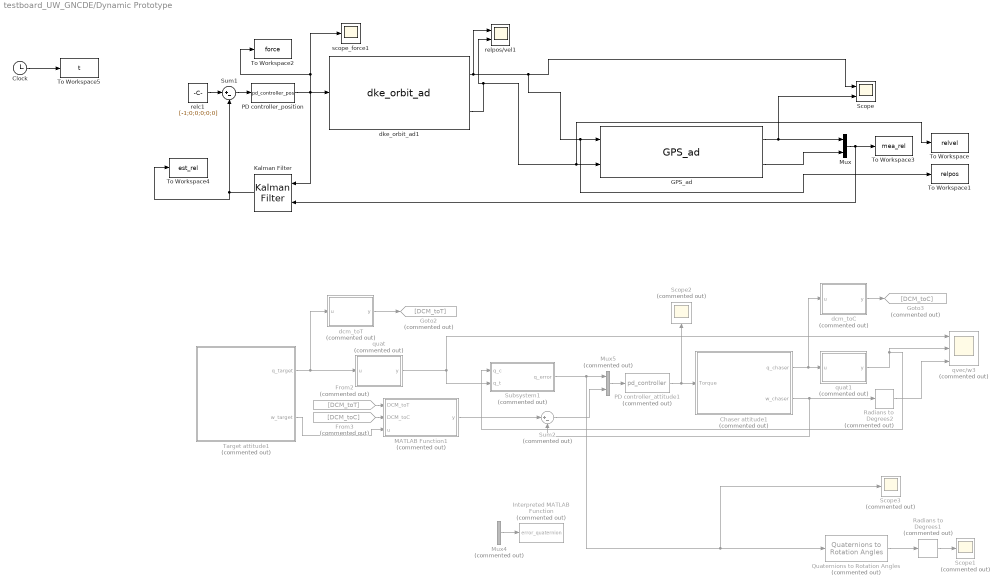
== system testboard_UW_GNCDE/Dynamic Prototype ==
  Chaser attitude1 : Subsystem  Commented=on
  Clock : Clock
  From2 : From  Commented=on  GotoTag=DCM_toT
  From3 : From  Commented=on  GotoTag=DCM_toC
  GPS_ad : GPS_ad/GPS_ad  DiagCtrlNo=6  Ini_option=Specify via Dialog  InitFileName=D:\GNCDE\working_folder\simulator\GPS_ad_init.m  NewFile_Action=Cancel  OldFile_Action=Cancel  InitStatus=off  GPS_ad_bias=[0,0,0,0,0,0]  GPS_ad_variance=[0.005,0.005,0.005,0.01,0.01,0.01]  GPS_ad_seed=[0,0,0,0,0,0]
  Goto2 : Goto  Commented=on  GotoTag=DCM_toT
  Goto3 : Goto  Commented=on  GotoTag=DCM_toC
  Interpreted MATLAB Function : MATLABFcn  Commented=on  MATLABFcn=error_quaternion
  Kalman Filter : ctrlSharedLib/Kalman Filter  TimeDomain=Continuous-Time  UseCurrentEstimator=on  ModelSource=Individual A, B, C, D matrices  ModelSourceVariable=sys  A=[zeros(3) eye(3); 0 0 0 0 0 0.002243; 0 -1.258e-6 0 0 0 0; 0 0 3.775e-6 -0.002243 0 0]  B=[zeros(3); 0.1*eye(3)]  C=[eye(6)]  D=[zeros(6,3)]  NumberOfStates=2  NumberOfInputs=2  NumberOfOutputs=2  InitialEstimateSource=Dialog  X0=[-5 0 0 0 0 0]  P0=10*eye(3,3)  UseK=off  UseGH=off  NumberOfProcessNoiseInputs=2  G=eye(6)  TimeInvariantG=on  H=100*eye(6)  TimeInvariantH=on  Q=0.05*eye(6)  TimeInvariantQ=on  R=0.001*eye(6)  TimeInvariantR=on  N=0  TimeInvariantN=on  AddInputPort=on  AddEnablePort=off  OutputEstimatedY=off  OutputP=off  Ts=0.01
      settings: SourceProductBaseCode=CT
  MATLAB Function1 : MATLAB Function  Commented=on  TreatAsAtomicUnit=on
  Mux : Mux  Inputs=2
  Mux4 : Mux  Commented=on  Inputs=2
  Mux5 : Mux  Commented=on  Inputs=2
  PD controller_attitude1 : MATLABFcn  Commented=on  MATLABFcn=pd_controller  OutputDimensions=3
  PD controller_position : MATLABFcn  MATLABFcn=pd_controller_pos  OutputDimensions=3
  Quaternions to Rotation Angles : sharedtransform/Quaternions to Rotation Angles  Commented=on  rotationOrder=ZYX  aMode=aMode
      settings: SourceProductBaseCode=AE
  Radians to Degrees1 : simulink_extras/Transformations/Radians to Degrees  Commented=on
  Radians to Degrees2 : simulink_extras/Transformations/Radians to Degrees  Commented=on
  Scope : Scope  NumInputPorts=2
  Scope1 : Scope  Commented=on
  Scope2 : Scope  Commented=on
  Scope3 : Scope  Commented=on
  Subsystem1 : Subsystem  Commented=on
  Sum1 : Sum  Inputs=|+-
  Sum2 : Sum  Commented=on  Inputs=|+-
  Target attitude1 : Subsystem  Commented=on
  To Workspace : ToWorkspace  VariableName=relvel  SaveFormat=Timeseries  SampleTime=-1
  To Workspace1 : ToWorkspace  VariableName=relpos  SaveFormat=Timeseries  SampleTime=-1
  To Workspace2 : ToWorkspace  VariableName=force  SaveFormat=Timeseries  SampleTime=-1
  To Workspace3 : ToWorkspace  VariableName=mea_rel  SaveFormat=Timeseries  SampleTime=-1
  To Workspace4 : ToWorkspace  VariableName=est_rel  SaveFormat=Timeseries  SampleTime=-1
  To Workspace5 : ToWorkspace  VariableName=t  SaveFormat=Timeseries  SampleTime=-1
  dcm_toC : MATLAB Function  Commented=on  TreatAsAtomicUnit=on
  dcm_toT : MATLAB Function  Commented=on  TreatAsAtomicUnit=on
  dke_orbit_ad1 : dke_orbit_ad/dke_orbit_ad  DiagCtrlNo=6  Ini_option=Specify via Dialog  InitFileName=D:\GNCDE\working_folder\simulator\dke_orbit_ad1_init.m  NewFile_Action=Cancel  OldFile_Action=Cancel  InitStatus=off  C_pos_rel_FT=[0,0,0]  C_vel_rel_FT=[0,0,0]  C_ini_pos_rel_FT=[-5;0;0]  C_ini_vel_rel_FT=[0;0;0.0839]  C_mass=10  T_orbital_rate=0.0011
  quat : MATLAB Function  Commented=on  TreatAsAtomicUnit=on
  quat1 : MATLAB Function  Commented=on  TreatAsAtomicUnit=on
  qvec/w3 : Scope  Commented=on  NumInputPorts=3
  relc1 : Constant  Value=[-1;0;0;0;0;0]
  relpos/vel1 : Scope  NumInputPorts=2
  scope_force1 : Scope
  wires:
  Sum1/1 -> PD controller_position/1
  relc1/1 -> Sum1/1
  dke_orbit_ad1/1 -> Scope/1, To Workspace1/1, GPS_ad/1, relpos/vel1/1
  dke_orbit_ad1/2 -> To Workspace/1, GPS_ad/2, relpos/vel1/2
  PD controller_position/1 -> Kalman Filter/1, dke_orbit_ad1/1, scope_force1/1, To Workspace2/1
  Kalman Filter/1 -> Sum1/2, To Workspace4/1
  GPS_ad/1 -> Scope/2, Mux/1
  GPS_ad/2 -> Mux/2
  Mux/1 -> Kalman Filter/2, To Workspace3/1
  Subsystem1/1(q_error) -> Quaternions to Rotation Angles/1, Scope3/1, Mux5/1
  Mux4/1 -> Interpreted MATLAB Function/1
  dcm_toC/1(y) -> Goto3/1
  dcm_toT/1(y) -> Goto2/1
  quat/1(y) -> Subsystem1/2(q_t), qvec/w3/1
  Quaternions to Rotation Angles/1 -> Radians to Degrees1/1
  Radians to Degrees2/1 -> qvec/w3/3
  Chaser attitude1/2(w_chaser) -> Radians to Degrees2/1, Sum2/2
  Mux5/1 -> PD controller_attitude1/1
  Target attitude1/1(q_target) -> dcm_toT/1(u), quat/1(u)
  Target attitude1/2(w_target) -> MATLAB Function1/3(u)
  Radians to Degrees1/1 -> Scope1/1
  Chaser attitude1/1(q_chaser) -> dcm_toC/1(u), quat1/1(u)
  From3/1 -> MATLAB Function1/2(DCM_toC)
  From2/1 -> MATLAB Function1/1(DCM_toT)
  MATLAB Function1/1(y) -> Sum2/1
  quat1/1(y) -> Subsystem1/1(q_c), qvec/w3/2
  PD controller_attitude1/1 -> Chaser attitude1/1(Torque), Scope2/1
  Sum2/1 -> Mux5/2
  Clock/1 -> To Workspace5/1
